simulink model "read_imu_data"  (R2022b)
settings: Solver=ode23t  StartTime=0.0  StopTime=90  MinStep=0.005  RelTol=1e-3
model workspace (MAT data in the model file):
  Logfile_Data_Object = robotics.ros.BagSelection
  Logfile_Data_Object.FilePath = '/home/tommaso/bags/gps_imu.bag'
  Logfile_Data_Object.StartTime = 1678126635.77
  Logfile_Data_Object.EndTime = 1678126731.34
  Logfile_Data_Object.NumMessages = 210047
  Logfile_Data_Object.AvailableTopics = table
  Logfile_Data_Object.AvailableTopics.data{1} = [19029; 19028; 500; 19031; 19035; 19030; 19035; 19029; 9514; 19030; 9516; 203; 19033; 19034]
  Logfile_Data_Object.AvailableTopics.data{2} = categorical
  Logfile_Data_Object.AvailableTopics.data{2}.categoryNames = {'geometry_msgs/QuaternionStamped'; 'geometry_msgs/Vector3Stamped'; 'rcl_interfaces/Log'; 'sensor_msgs/FluidPressure'; 'sensor_msgs/Imu'; 'sensor_msgs/MagneticField'; 'sensor_msgs/NavSatFix'; 'sensor_msgs/Temperature'; 'sensor_msgs/TimeReference'; 'tf2_msgs/TFMessage'}
  Logfile_Data_Object.AvailableTopics.data{2}.codes = [2; 1; 7; 2; 2; 5; 1; 2; 6; 9; 4; 3; 8; 10]
  Logfile_Data_Object.AvailableTopics.data{3}{1} = 'std_msgs/Header Header
    |   uint32 Seq
    |   Time Stamp
    |   char FrameId
    | geometry_msgs/Vector3 Vector
    |   double X
    |   double Y
    |   double Z
    | '
  Logfile_Data_Object.AvailableTopics.data{3}{2} = 'std_msgs/Header Header
    |   uint32 Seq
    |   Time Stamp
    |   char FrameId
    | geometry_msgs/Quaternion Quaternion
    |   double X
    |   double Y
    |   double Z
    |   double W
    | '
  Logfile_Data_Object.AvailableTopics.data{3}{3} = 'uint8 COVARIANCETYPEUNKNOWN
    | uint8 COVARIANCETYPEAPPROXIMATED
    | uint8 COVARIANCETYPEDIAGONALKNOWN
    | uint8 COVARIANCETYPEKNOWN
    | std_msgs/Header Header
    |   uint32 Seq
    |   Time Stamp
    |   char FrameId
    | sensor_msgs/NavSatStatus Status
    |   int8 STATUSNOFIX
    |   int8 STATUSFIX
    |   int8 STATUSSBASFIX
    |   int8 STATUSGBASFIX
    |   uint16 SERVICEGPS
    |   uint16 SERVICEGLONASS
    |   uint16 SERVICECOMPASS
    |   uint16 SERVICEGALILEO
    |   int8 Status
    |   uint16 Service
    | double Latitude
    | double Longitude
    | double Altitude
    | double[9] PositionCovariance
    | uint8 PositionCovarianceType
    | '
  Logfile_Data_Object.AvailableTopics.data{3}{4} = 'std_msgs/Header Header
    |   uint32 Seq
    |   Time Stamp
    |   char FrameId
    | geometry_msgs/Vector3 Vector
    |   double X
    |   double Y
    |   double Z
    | '
  Logfile_Data_Object.AvailableTopics.data{3}{5} = 'std_msgs/Header Header
    |   uint32 Seq
    |   Time Stamp
    |   char FrameId
    | geometry_msgs/Vector3 Vector
    |   double X
    |   double Y
    |   double Z
    | '
  Logfile_Data_Object.AvailableTopics.data{3}{6} = 'std_msgs/Header Header
    |   uint32 Seq
    |   Time Stamp
    |   char FrameId
    | geometry_msgs/Quaternion Orientation
    |   double X
    |   double Y
    |   double Z
    |   double W
    | double[9] OrientationCovariance
    | geometry_msgs/Vector3 AngularVelocity
    |   double X
    |   double Y
    |   double Z
    | double[9] AngularVelocityCovariance
    | geometry_msgs/Vector3 LinearAcceleration
    |   double X
    |   double Y
    |   double Z
    | double[9] LinearAccelerationCovariance
    | '
  Logfile_Data_Object.AvailableTopics.data{3}{7} = 'std_msgs/Header Header
    |   uint32 Seq
    |   Time Stamp
    |   char FrameId
    | geometry_msgs/Quaternion Quaternion
    |   double X
    |   double Y
    |   double Z
    |   double W
    | '
  Logfile_Data_Object.AvailableTopics.data{3}{8} = 'std_msgs/Header Header
    |   uint32 Seq
    |   Time Stamp
    |   char FrameId
    | geometry_msgs/Vector3 Vector
    |   double X
    |   double Y
    |   double Z
    | '
  Logfile_Data_Object.AvailableTopics.data{3}{9} = 'std_msgs/Header Header
    |   uint32 Seq
    |   Time Stamp
    |   char FrameId
    | geometry_msgs/Vector3 MagneticField
    |   double X
    |   double Y
    |   double Z
    | double[9] MagneticFieldCovariance
    | '
  Logfile_Data_Object.AvailableTopics.data{3}{10} = 'std_msgs/Header Header
    |   uint32 Seq
    |   Time Stamp
    |   char FrameId
    | Time TimeRef
    | char Source
    | '
  Logfile_Data_Object.AvailableTopics.data{3}{11} = 'std_msgs/Header Header
    |   uint32 Seq
    |   Time Stamp
    |   char FrameId
    | double FluidPressure
    | double Variance
    | '
  Logfile_Data_Object.AvailableTopics.data{3}{12} = 'uint8 DEBUG
    | uint8 INFO
    | uint8 WARN
    | uint8 ERROR
    | uint8 FATAL
    | Time Stamp
    | uint8 Level
    | char Name
    | char Msg
    | char File
    | char Function
    | uint32 Line
    | '
  Logfile_Data_Object.AvailableTopics.data{3}{13} = 'std_msgs/Header Header
    |   uint32 Seq
    |   Time Stamp
    |   char FrameId
    | double Temperature
    | double Variance
    | '
  Logfile_Data_Object.AvailableTopics.data{3}{14} = 'geometry_msgs/TransformStamped[] Transforms
    |   std_msgs/Header Header
    |     uint32 Seq
    |     Time Stamp
    |     char FrameId
    |   char ChildFrameId
    |   geometry_msgs/Transform Transform
    |     geometry_msgs/Vector3 Translation
    |       double X
    |       double Y
    |       double Z
    |     geometry_msgs/Quaternion Rotation
    |       double X
    |       double Y
    |       double Z
    |       double W
    | '
  Logfile_Data_Object.AvailableTopics.ndims = 2
  Logfile_Data_Object.AvailableTopics.nrows = 14
  Logfile_Data_Object.AvailableTopics.rownames = {'/filter/free_acceleration'; '/filter/quaternion'; '/gps/position'; '/imu/acceleration'; '/imu/angular_velocity'; '/imu/data'; '/imu/dq'; '/imu/dv'; '/imu/mag'; '/imu/time_ref'; '/pressure'; '/rosout'; '/temperature'; '/tf'}
  Logfile_Data_Object.AvailableTopics.nvars = 3
  Logfile_Data_Object.AvailableTopics.varnames = {'NumMessages', 'MessageType', 'MessageDefinition'}
  Logfile_Data_Object.AvailableTopics.props.useVariableNamesOriginal = 0
  Logfile_Data_Object.AvailableTopics.props.useDimensionNamesOriginal = 0
  Logfile_Data_Object.AvailableTopics.props.CustomProps = struct()
  Logfile_Data_Object.AvailableTopics.props.VariableCustomProps = struct()
  Logfile_Data_Object.AvailableTopics.props.versionSavedFrom = 4
  Logfile_Data_Object.AvailableTopics.props.minCompatibleVersion = 1
  Logfile_Data_Object.AvailableTopics.props.incompatibilityMsg = ''
  Logfile_Data_Object.AvailableTopics.props.VersionSavedFrom = 4
  Logfile_Data_Object.AvailableTopics.props.Description = ''
  Logfile_Data_Object.AvailableTopics.props.VariableNamesOriginal = {}
  Logfile_Data_Object.AvailableTopics.props.DimensionNames = {'Row', 'Variables'}
  Logfile_Data_Object.AvailableTopics.props.DimensionNamesOriginal = {}
  Logfile_Data_Object.AvailableTopics.props.UserData = []
  Logfile_Data_Object.AvailableTopics.props.VariableDescriptions = {}
  Logfile_Data_Object.AvailableTopics.props.VariableUnits = {}
  Logfile_Data_Object.AvailableTopics.props.VariableContinuity = {}
  Logfile_Data_Object.AvailableFrames = {'imu_link'; 'world'}
  Logfile_Data_Object.MessageList = table
  Logfile_Data_Object.MessageList.data{1} = [1678126635.77 1678126635.77 1678126635.77 1678126635.77 1678126635.77 1678126635.77 1678126635.77 1678126635.77 1678126635.77 1678126635.77 1678126635.77 1678126636.16 ... (210047 elements, 210047x1)]
  Logfile_Data_Object.MessageList.data{2} = categorical
  Logfile_Data_Object.MessageList.data{2}.categoryNames = {'/filter/free_acceleration'; '/filter/quaternion'; '/gps/position'; '/imu/acceleration'; '/imu/angular_velocity'; '/imu/data'; '/imu/dq'; '/imu/dv'; '/imu/mag'; '/imu/time_ref'; '/pressure'; '/rosout'; '/temperature'; '/tf'}
  Logfile_Data_Object.MessageList.data{2}.codes = [12 12 12 12 12 12 12 12 12 12 12 12 ... (210047 elements, 210047x1)]
  Logfile_Data_Object.MessageList.data{3} = categorical
  Logfile_Data_Object.MessageList.data{3}.categoryNames = {'geometry_msgs/Vector3Stamped'; 'geometry_msgs/QuaternionStamped'; 'sensor_msgs/NavSatFix'; 'sensor_msgs/Imu'; 'sensor_msgs/MagneticField'; 'sensor_msgs/TimeReference'; 'sensor_msgs/FluidPressure'; 'rcl_interfaces/Log'; 'sensor_msgs/Temperature'; 'tf2_msgs/TFMessage'}
  Logfile_Data_Object.MessageList.data{3}.codes = [8 8 8 8 8 8 8 8 8 8 8 8 ... (210047 elements, 210047x1)]
  Logfile_Data_Object.MessageList.data{4} = [15754 15976 16204 16426 16654 16876 17104 17326 17554 17776 18004 18226 ... (210047 elements, 210047x1)]
  Logfile_Data_Object.MessageList.ndims = 2
  Logfile_Data_Object.MessageList.nrows = 210047
  Logfile_Data_Object.MessageList.nvars = 4
  Logfile_Data_Object.MessageList.varnames = {'Time', 'Topic', 'MessageType', 'FileOffset'}
  Logfile_Data_Object.MessageList.props.useVariableNamesOriginal = 0
  Logfile_Data_Object.MessageList.props.useDimensionNamesOriginal = 0
  Logfile_Data_Object.MessageList.props.CustomProps = struct()
  Logfile_Data_Object.MessageList.props.VariableCustomProps = struct()
  Logfile_Data_Object.MessageList.props.versionSavedFrom = 4
  Logfile_Data_Object.MessageList.props.minCompatibleVersion = 1
  Logfile_Data_Object.MessageList.props.incompatibilityMsg = ''
  Logfile_Data_Object.MessageList.props.VersionSavedFrom = 4
  Logfile_Data_Object.MessageList.props.Description = ''
  Logfile_Data_Object.MessageList.props.VariableNamesOriginal = {}
  Logfile_Data_Object.MessageList.props.DimensionNames = {'Row', 'Variables'}
  Logfile_Data_Object.MessageList.props.DimensionNamesOriginal = {}
  Logfile_Data_Object.MessageList.props.UserData = []
  Logfile_Data_Object.MessageList.props.VariableDescriptions = {}
  Logfile_Data_Object.MessageList.props.VariableUnits = {}
  Logfile_Data_Object.MessageList.props.VariableContinuity = {}
  Logfile_Data_Object.RawMessageBuffer = containers.Map
  Logfile_Data_Object.RawMessageBuffer.serialization.keys = {}
  Logfile_Data_Object.RawMessageBuffer.serialization.values = {}
  Logfile_Data_Object.RawMessageBuffer.serialization.uniformity = 0
  Logfile_Data_Object.RawMessageBuffer.serialization.keyType = 'char'
  Logfile_Data_Object.RawMessageBuffer.serialization.valueType = 'any'
  Logfile_Data_Object.ImgMessageBuffer = containers.Map
  Logfile_Data_Object.ImgMessageBuffer.serialization.keys = {}
  Logfile_Data_Object.ImgMessageBuffer.serialization.values = {}
  Logfile_Data_Object.ImgMessageBuffer.serialization.uniformity = 0
  Logfile_Data_Object.ImgMessageBuffer.serialization.keyType = 'char'
  Logfile_Data_Object.ImgMessageBuffer.serialization.valueType = 'any'
  Logfile_Data_Object.TopicTypeMap = containers.Map
  Logfile_Data_Object.TopicTypeMap.serialization.keys = {'/filter/free_acceleration', '/filter/quaternion', '/gps/position', '/imu/acceleration', '/imu/angular_velocity', '/imu/data', '/imu/dq', '/imu/dv', '/imu/mag', '/imu/time_ref', '/pressure', '/rosout', '/temperature', '/tf'}
  Logfile_Data_Object.TopicTypeMap.serialization.values = {'geometry_msgs/Vector3Stamped', 'geometry_msgs/QuaternionStamped', 'sensor_msgs/NavSatFix', 'geometry_msgs/Vector3Stamped', 'geometry_msgs/Vector3Stamped', 'sensor_msgs/Imu', 'geometry_msgs/QuaternionStamped', 'geometry_msgs/Vector3Stamped', 'sensor_msgs/MagneticField', 'sensor_msgs/TimeReference', 'sensor_msgs/FluidPressure', 'rcl_interfaces/Log', 'sensor_msgs/Temperature', 'tf2_msgs/TFMessage'}
  Logfile_Data_Object.TopicTypeMap.serialization.uniformity = 1
  Logfile_Data_Object.TopicTypeMap.serialization.keyType = 'char'
  Logfile_Data_Object.TopicTypeMap.serialization.valueType = 'char'
  Logfile_Data_Object.TopicDefinitionMap = containers.Map
  Logfile_Data_Object.TopicDefinitionMap.serialization.keys = {'/filter/free_acceleration', '/filter/quaternion', '/gps/position', '/imu/acceleration', '/imu/angular_velocity', '/imu/data', '/imu/dq', '/imu/dv', '/imu/mag', '/imu/time_ref', '/pressure', '/rosout', '/temperature', '/tf'}
  Logfile_Data_Object.TopicDefinitionMap.serialization.values{1} = 'std_msgs/Header Header
    |   uint32 Seq
    |   Time Stamp
    |   char FrameId
    | geometry_msgs/Vector3 Vector
    |   double X
    |   double Y
    |   double Z
    | '
  Logfile_Data_Object.TopicDefinitionMap.serialization.values{2} = 'std_msgs/Header Header
    |   uint32 Seq
    |   Time Stamp
    |   char FrameId
    | geometry_msgs/Quaternion Quaternion
    |   double X
    |   double Y
    |   double Z
    |   double W
    | '
  Logfile_Data_Object.TopicDefinitionMap.serialization.values{3} = 'uint8 COVARIANCETYPEUNKNOWN
    | uint8 COVARIANCETYPEAPPROXIMATED
    | uint8 COVARIANCETYPEDIAGONALKNOWN
    | uint8 COVARIANCETYPEKNOWN
    | std_msgs/Header Header
    |   uint32 Seq
    |   Time Stamp
    |   char FrameId
    | sensor_msgs/NavSatStatus Status
    |   int8 STATUSNOFIX
    |   int8 STATUSFIX
    |   int8 STATUSSBASFIX
    |   int8 STATUSGBASFIX
    |   uint16 SERVICEGPS
    |   uint16 SERVICEGLONASS
    |   uint16 SERVICECOMPASS
    |   uint16 SERVICEGALILEO
    |   int8 Status
    |   uint16 Service
    | double Latitude
    | double Longitude
    | double Altitude
    | double[9] PositionCovariance
    | uint8 PositionCovarianceType
    | '
  Logfile_Data_Object.TopicDefinitionMap.serialization.values{4} = 'std_msgs/Header Header
    |   uint32 Seq
    |   Time Stamp
    |   char FrameId
    | geometry_msgs/Vector3 Vector
    |   double X
    |   double Y
    |   double Z
    | '
  Logfile_Data_Object.TopicDefinitionMap.serialization.values{5} = 'std_msgs/Header Header
    |   uint32 Seq
    |   Time Stamp
    |   char FrameId
    | geometry_msgs/Vector3 Vector
    |   double X
    |   double Y
    |   double Z
    | '
  Logfile_Data_Object.TopicDefinitionMap.serialization.values{6} = 'std_msgs/Header Header
    |   uint32 Seq
    |   Time Stamp
    |   char FrameId
    | geometry_msgs/Quaternion Orientation
    |   double X
    |   double Y
    |   double Z
    |   double W
    | double[9] OrientationCovariance
    | geometry_msgs/Vector3 AngularVelocity
    |   double X
    |   double Y
    |   double Z
    | double[9] AngularVelocityCovariance
    | geometry_msgs/Vector3 LinearAcceleration
    |   double X
    |   double Y
    |   double Z
    | double[9] LinearAccelerationCovariance
    | '
  Logfile_Data_Object.TopicDefinitionMap.serialization.values{7} = 'std_msgs/Header Header
    |   uint32 Seq
    |   Time Stamp
    |   char FrameId
    | geometry_msgs/Quaternion Quaternion
    |   double X
    |   double Y
    |   double Z
    |   double W
    | '
  Logfile_Data_Object.TopicDefinitionMap.serialization.values{8} = 'std_msgs/Header Header
    |   uint32 Seq
    |   Time Stamp
    |   char FrameId
    | geometry_msgs/Vector3 Vector
    |   double X
    |   double Y
    |   double Z
    | '
  Logfile_Data_Object.TopicDefinitionMap.serialization.values{9} = 'std_msgs/Header Header
    |   uint32 Seq
    |   Time Stamp
    |   char FrameId
    | geometry_msgs/Vector3 MagneticField
    |   double X
    |   double Y
    |   double Z
    | double[9] MagneticFieldCovariance
    | '
  Logfile_Data_Object.TopicDefinitionMap.serialization.values{10} = 'std_msgs/Header Header
    |   uint32 Seq
    |   Time Stamp
    |   char FrameId
    | Time TimeRef
    | char Source
    | '
  Logfile_Data_Object.TopicDefinitionMap.serialization.values{11} = 'std_msgs/Header Header
    |   uint32 Seq
    |   Time Stamp
    |   char FrameId
    | double FluidPressure
    | double Variance
    | '
  Logfile_Data_Object.TopicDefinitionMap.serialization.values{12} = 'uint8 DEBUG
    | uint8 INFO
    | uint8 WARN
    | uint8 ERROR
    | uint8 FATAL
    | Time Stamp
    | uint8 Level
    | char Name
    | char Msg
    | char File
    | char Function
    | uint32 Line
    | '
  Logfile_Data_Object.TopicDefinitionMap.serialization.values{13} = 'std_msgs/Header Header
    |   uint32 Seq
    |   Time Stamp
    |   char FrameId
    | double Temperature
    | double Variance
    | '
  Logfile_Data_Object.TopicDefinitionMap.serialization.values{14} = 'geometry_msgs/TransformStamped[] Transforms
    |   std_msgs/Header Header
    |     uint32 Seq
    |     Time Stamp
    |     char FrameId
    |   char ChildFrameId
    |   geometry_msgs/Transform Transform
    |     geometry_msgs/Vector3 Translation
    |       double X
    |       double Y
    |       double Z
    |     geometry_msgs/Quaternion Rotation
    |       double X
    |       double Y
    |       double Z
    |       double W
    | '
  Logfile_Data_Object.TopicDefinitionMap.serialization.uniformity = 1
  Logfile_Data_Object.TopicDefinitionMap.serialization.keyType = 'char'
  Logfile_Data_Object.TopicDefinitionMap.serialization.valueType = 'char'
  Logfile_Data_Object.messageTypeMap = containers.Map
  Logfile_Data_Object.messageTypeMap.serialization.keys = {}
  Logfile_Data_Object.messageTypeMap.serialization.values = {}
  Logfile_Data_Object.messageTypeMap.serialization.uniformity = 0
  Logfile_Data_Object.messageTypeMap.serialization.keyType = 'char'
  Logfile_Data_Object.messageTypeMap.serialization.valueType = 'any'
  Logfile_Data_Object.Parser = robotics.ros.internal.tf.TransformationTreeParser
  Logfile_Data_Object.Parser.UseObjectMsg = 1
  Logfile_Path = '/home/tommaso/bags/gps_imu.bag'
  Logfile_Playback_Duration = nan
  Logfile_Playback_Offset = 1
libraries: robotlib x2
settings Model: SimulationMode=accelerator  Creator=The MathWorks, Inc.  LastModifiedBy=tommaso
settings SolverCC: AlgebraicLoopSolver=TrustRegion
settings DataIOCC: ReturnWorkspaceOutputs=off
settings DebuggingCC: UnconnectedInputMsg=warning  UnconnectedOutputMsg=warning  UnconnectedLineMsg=warning  SFMachineParentedDataDiag=warning  ArithmeticOperatorsInVariantConditions=warning
settings ModelReferenceCC: EnableRefExpFcnMdlSchedulingChecks=on
settings RTWCC: DLArmComputeVersion=19.05

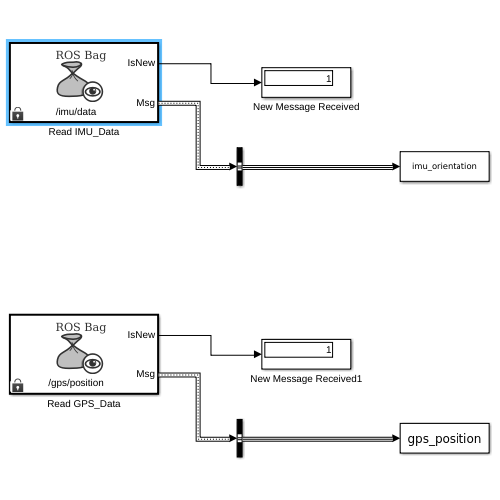
[thumbnail: Simulink's stored preview of the top-level diagram]
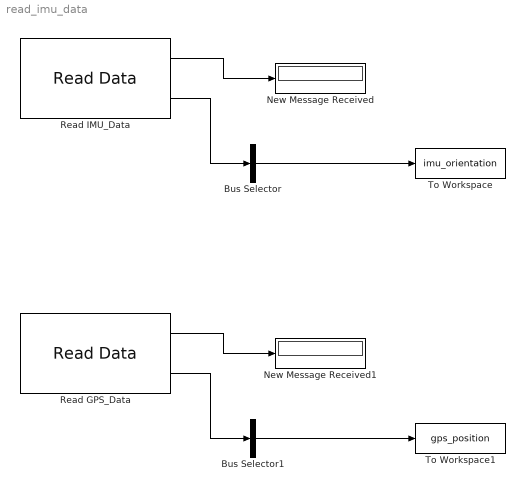
== system read_imu_data ==
  Bus Selector : BusSelector  OutputSignals=Orientation,AngularVelocity,LinearAcceleration,AngularVelocityCovariance,LinearAccelerationCovariance  OutputAsBus=on
  Bus Selector1 : BusSelector  OutputSignals=Latitude,Longitude,Altitude,PositionCovariance,PositionCovarianceType  OutputAsBus=on
  New Message Received : Display
  New Message Received1 : Display
  Read GPS_Data : robotlib/Read Data  topic=/gps/position  sampleTime=1  logfileType=rosbag  modelName=read_imu_data  msgType=sensor_msgs/NavSatFix
      settings: LibrarySourceBlock=roslib/ROS/Read Data
  Read IMU_Data : robotlib/Read Data  topic=/imu/data  sampleTime=0.005  logfileType=rosbag  modelName=read_imu_data  msgType=sensor_msgs/Imu
      settings: LibrarySourceBlock=roslib/ROS/Read Data
  To Workspace : ToWorkspace  VariableName=imu_orientation  SaveFormat=Timeseries  SampleTime=-1
  To Workspace1 : ToWorkspace  VariableName=gps_position  SaveFormat=Timeseries  SampleTime=-1
  wires:
  Read IMU_Data/2 -> Bus Selector/1
  Read IMU_Data/1 -> New Message Received/1
  Bus Selector/1 -> To Workspace/1
  Read GPS_Data/2 -> Bus Selector1/1
  Read GPS_Data/1 -> New Message Received1/1
  Bus Selector1/1 -> To Workspace1/1
